simulink model "regPIsim"  (R2022b)
settings: Solver=VariableStepAuto  StartTime=0.0  StopTime=t  MaxStep=maxStep  RelTol=1e-3
values from neighbouring files (symbols this model uses):
  k = ki(i)    [regPI.m]    (also in regulator.m = kp(i))
  kp = 5    [regPI.m]    (also in regulator.m = linspace(0.5*Kp,0.8*Kp,4))
settings Model: Creator=wojna  LastModifiedBy=wojna

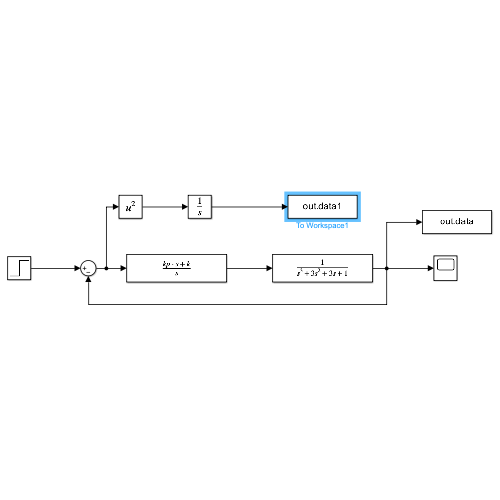
[thumbnail: Simulink's stored preview of the top-level diagram]
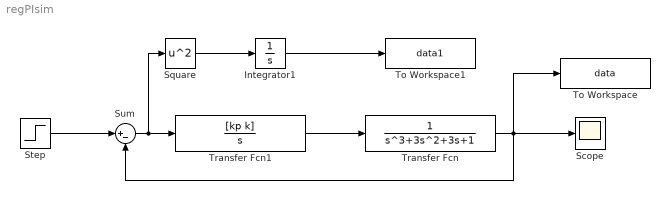
== system regPIsim ==
  Integrator1 : Integrator
  Scope : Scope
  Square : Math  Operator=square
  Step : Step  SampleTime=0
  Sum : Sum  Inputs=|+-
  To Workspace : ToWorkspace  VariableName=data  SaveFormat=Timeseries  SampleTime=-1
  To Workspace1 : ToWorkspace  VariableName=data1  SaveFormat=Timeseries  SampleTime=-1
  Transfer Fcn : TransferFcn  Denominator=[1 3 3 1]
  Transfer Fcn1 : TransferFcn  Numerator=[kp k]  Denominator=[1 0]
  wires:
  Transfer Fcn1/1 -> Transfer Fcn/1
  Transfer Fcn/1 -> To Workspace/1, Scope/1, Sum/2
  Sum/1 -> Transfer Fcn1/1, Square/1
  Step/1 -> Sum/1
  Square/1 -> Integrator1/1
  Integrator1/1 -> To Workspace1/1
